simulink model "week2_que1"  (R2020b)
settings: Solver=VariableStepAuto  StartTime=0.0  StopTime=inf  RelTol=1e-3
libraries: simulink_extras x3
settings Model: Creator=mluser  LastModifiedBy=mluser

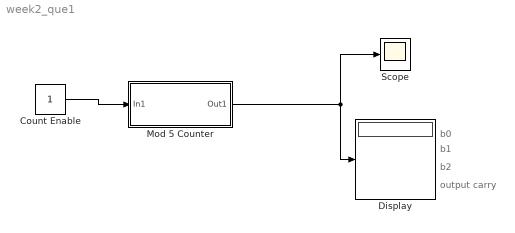
== system week2_que1 ==
  note: output carry
  note: b2
  note: b1
  note: b0
  Count Enable : Constant  OutDataTypeStr=boolean
  Display : Display
  Mod 5 Counter : Subsystem
  Scope : Scope
  wires:
  Count Enable/1 -> Mod 5 Counter/1(In1)
  Mod 5 Counter/1(Out1) -> Display/1, Scope/1

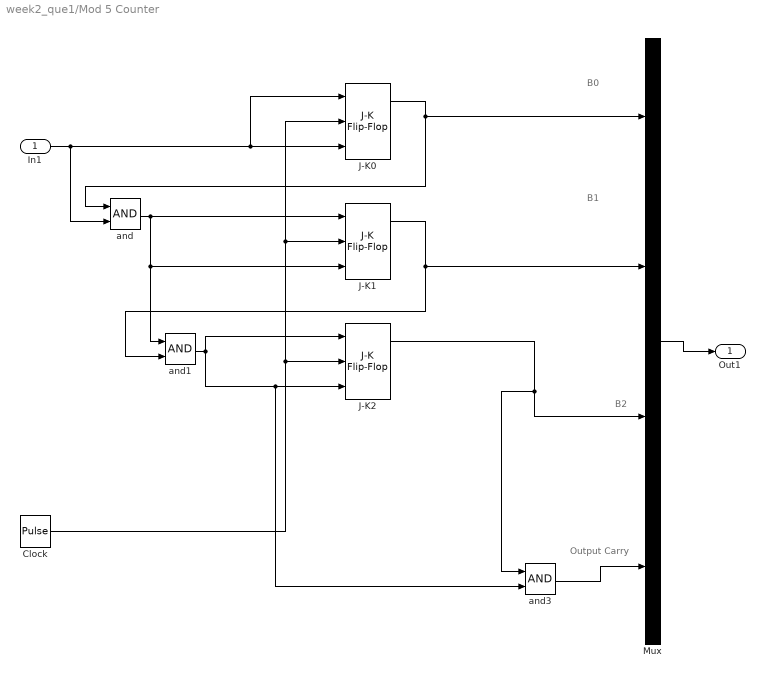
== system week2_que1/Mod 5 Counter ==
  note: B1
  note: B0
  note: B2
  note: Output Carry
  In1 : Inport
  Clock : DiscretePulseGenerator  PulseType=Time based  Period=1  PhaseDelay=1
  J-K0 : simulink_extras/Flip Flops/J-K Flip-Flop  initial_condition=0
  J-K1 : simulink_extras/Flip Flops/J-K Flip-Flop  initial_condition=0
  J-K2 : simulink_extras/Flip Flops/J-K Flip-Flop  initial_condition=0
  Mux : Mux
  and : Logic  AllPortsSameDT=off  OutDataTypeStr=boolean
  and1 : Logic  AllPortsSameDT=off  OutDataTypeStr=boolean
  and3 : Logic  AllPortsSameDT=off  OutDataTypeStr=boolean
  Out1 : Outport
  wires:
  and/1 -> J-K1/1, and1/1, J-K1/3
  J-K2/1 -> and3/1, Mux/3
  J-K0/1 -> and/1, Mux/1
  and1/1 -> J-K2/1, and3/2, J-K2/3
  and3/1 -> Mux/4
  In1/1 -> J-K0/3, J-K0/1, and/2
  J-K1/1 -> and1/2, Mux/2
  Clock/1 -> J-K0/2, J-K1/2, J-K2/2
  Mux/1 -> Out1/1
